simulink model "TP2_R3FOCPuente_ctrl_2016"  (R2016a)
settings: Solver=ode15s  StartTime=0.0  StopTime=.2  FixedStep=1e-6  RelTol=1e-5
values from neighbouring files (symbols this model uses):
  t1 = fase1+theta    (= 0.005)    [TP2_R3FMO_ctrl_2016.m]    (also in TP2_R3FMO_ctrl_2016_p_2.m; TP2_R3FMO_ctrl_2016_p_3.m)
  t2 = fase2+theta    (= 0.0116666666667)    [TP2_R3FMO_ctrl_2016.m]    (also in TP2_R3FMO_ctrl_2016_p_2.m; TP2_R3FMO_ctrl_2016_p_3.m)
  t3 = fase3+theta    (= 0.0183333333333)    [TP2_R3FMO_ctrl_2016.m]    (also in TP2_R3FMO_ctrl_2016_p_2.m; TP2_R3FMO_ctrl_2016_p_3.m)
undefined symbols (not defined in the file or in its folder): d
libraries: powerlib x21, powerlib_meascontrol x1
settings Model: Creator=Monina  LastModifiedBy=bress
settings DataIOCC: SaveFormat=Array  SignalLoggingSaveFormat=ModelDataLogs  TimeSaveName=t
settings OptimizationCC: ExpressionDepthLimit=2147483647
settings DebuggingCC: UnderspecifiedInitializationDetection=Classic  MergeDetectMultiDrivingBlocksExec=none  SolverPrmCheckMsg=warning  FcnCallInpInsideContextMsg=EnableAllAsWarning  StateNameClashWarn=warning
settings HardwareCC: ProdBitPerPointer=32  ProdLargestAtomicFloat=None  ProdIntDivRoundTo=Undefined  ProdEndianess=Unspecified  ProdWordSize=32  ProdHWDeviceType=32-bit Generic
settings ModelReferenceCC: PropagateSignalLabelsOutOfModel=off
settings GRTTargetCC: CombineOutputUpdateFcns=off  GRTInterface=on
settings ConfigComp: CovSFcnEnable=off
settings SimscapeCC: SimscapeNormalizeSystem=off

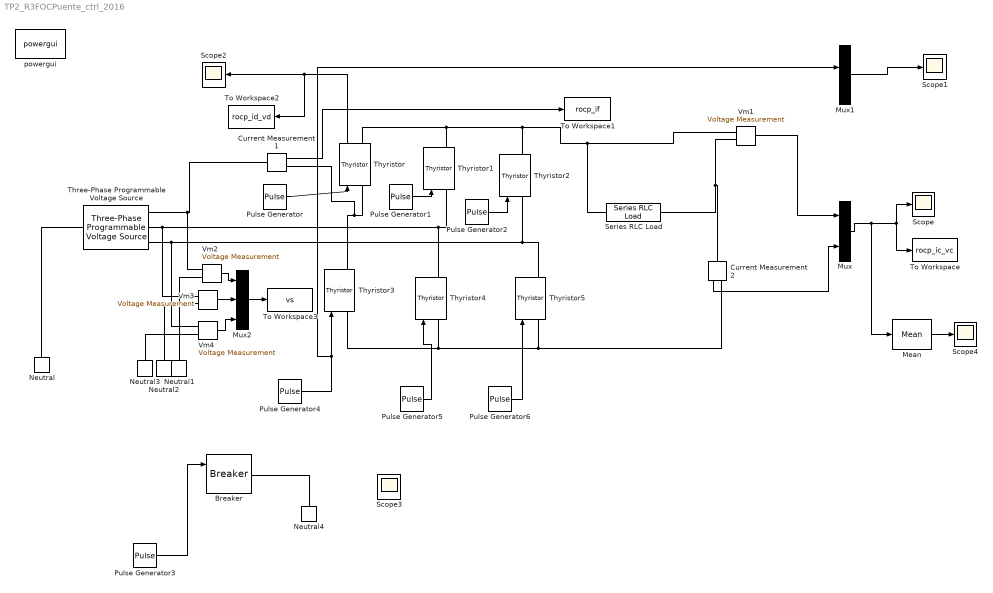
== system TP2_R3FOCPuente_ctrl_2016 ==
  Breaker : powerlib/Elements/Breaker  InitialState=0  SwitchingTimes="[1/60  5/60]"  External=on  BreakerResistance=0.01  SnubberResistance=1e6  SnubberCapacitance=inf  Measurements=None  MoreParameters=on  NoBreakLoop=off
  Current Measurement1 : powerlib/Measurements/Current Measurement  PhasorSimulation=off  OutputType=Complex  PSBequivalent=0
  Current Measurement2 : powerlib/Measurements/Current Measurement  PhasorSimulation=off  OutputType=Complex  PSBequivalent=0
  Mean : powerlib_meascontrol/Measurements/Mean  Freq=50  Vinit=0  Ts=0
  Mux : Mux  Inputs=2
  Mux1 : Mux
  Mux2 : Mux  Inputs=3
  Neutral{,1..4} (5 alike) : powerlib/Elements/Neutral  LConnTagsString=a  NodeNumber=10
  Pulse Generator : DiscretePulseGenerator  PulseType=Time based  Period=.02  PulseWidth=d  PhaseDelay=t1
  Pulse Generator1 : DiscretePulseGenerator  PulseType=Time based  Period=.02  PulseWidth=d  PhaseDelay=t2
  Pulse Generator2 : DiscretePulseGenerator  PulseType=Time based  Period=.02  PulseWidth=d  PhaseDelay=t3
  Pulse Generator3 : DiscretePulseGenerator  PulseType=Time based  Period=10  PulseWidth=50  PhaseDelay=.5
  Pulse Generator4 : DiscretePulseGenerator  PulseType=Time based  Period=.02  PulseWidth=d  PhaseDelay=t1+.01
  Pulse Generator5 : DiscretePulseGenerator  PulseType=Time based  Period=.02  PulseWidth=d  PhaseDelay=t2+.01
  Pulse Generator6 : DiscretePulseGenerator  PulseType=Time based  Period=.02  PulseWidth=d  PhaseDelay=t3+.01
  Scope{,1..4} (5 alike) : Scope
  Series RLC Load : powerlib/Elements/Series RLC Load  LConnTagsString=a  RConnTagsString=__new0  NominalVoltage=220  NominalFrequency=50  ActivePower=5000  InductivePower=500  CapacitivePower=0  Setx0=off  InitialVoltage=0  SetiL0=off  InitialCurrent=0  Measurements=None  LoadType=constant Z
  Three-Phase Programmable Voltage Source : powerlib/Electrical Sources/Three-Phase Programmable Voltage Source  PositiveSequence="[380  0 50]"  VariationEntity=None  VariationType=Table of time-amplitude pairs  VariationTypeAlt=Step  VariationStep=0.5  VariationRate=10  VariationMagnitude=0.3  VariationFrequency=2  VariationTiming=[1 2]  VariationPhaseA=off  Amplitudes=[1 0.8 1.2 1.0]  TimeValues=[0 0.1 0.15 0.2]  HarmonicGeneration=off  HarmonicA=[3 0.2 -25 0]  HarmonicB=[2 0.15 35 2]  Timing="[0.05  3]"  BusType=swing  Pref=0  Qref=0  Qmin=-inf  Qmax=inf
  Thyristor{,1..5} (6 alike) : powerlib/Power Electronics/Thyristor  Ron=0.001  Lon=0  Vf=0.8  IC=0  Rs=400  Cs=500e-10  Measurements=on
  To Workspace : ToWorkspace  VariableName=rocp_ic_vc  SampleTime=-1
  To Workspace1 : ToWorkspace  VariableName=rocp_if  SampleTime=-1
  To Workspace2 : ToWorkspace  VariableName=rocp_id_vd  SampleTime=-1
  To Workspace3 : ToWorkspace  VariableName=vs  SampleTime=-1
  Vm{1..4} (4 alike) : powerlib/Measurements/Voltage Measurement  PhasorSimulation=off  OutputType=Complex  PSBequivalent=0
  powergui : powerlib/powergui  Priority=1  SimulationMode=Continuous  SampleTime=50e-6  frequency=60  Iterations=50  frequencyindice=50  Pbase=100e6  ErrMax=1e-4  UnitsV=kV  UnitsW=MW  buscounter=0  FunctionMessages=off  echomessages=off  EnableUseOfTLC=off  CurrentSourceSwitches=on  DisableSnubberDevices=off  DisableRonSwitches=off  DisableVfSwitches=off  DisplayEquations=off  SolverType=Tustin  Interpol=off  ExternalGateDelay=off  methode=off  Ts=0  x0status=blocks  SPID=off  SwTol=0  HookPort=off  RestoreLinks=warning  ResistiveCurrentMeasurement=off  Frange=[0:2:500]  Ylog=off  Xlog=on  ShowGrid=off  save=off  variable=ZData  structure=0  ZoomFFT=off  StartTime=0.0  cycles=1  DisplayStyle=1  fundamental=60  FreqAxis=off  MaxFrequency=1000  frequencyindicesteady=1  RmsSteady=1  display=off
  wires:
  Mux/1 -> Mean/1, Scope/1, To Workspace/1
  Current Measurement1/1 -> To Workspace1/1
  Thyristor/1 -> To Workspace2/1, Scope2/1
  Mux1/1 -> Scope1/1
  Current Measurement2/1 -> Mux/2
  Pulse Generator/1 -> Thyristor/1
  Pulse Generator1/1 -> Thyristor1/1
  Pulse Generator2/1 -> Thyristor2/1
  Vm2/1 -> Mux2/1
  Vm3/1 -> Mux2/2
  Vm4/1 -> Mux2/3
  Mux2/1 -> To Workspace3/1
  Vm1/1 -> Mux/1
  Mean/1 -> Scope4/1
  Pulse Generator3/1 -> Breaker/1
  Pulse Generator4/1 -> Mux1/2, Thyristor3/1
  Pulse Generator5/1 -> Thyristor4/1
  Pulse Generator6/1 -> Thyristor5/1
  connections:
  Three-Phase Programmable Voltage Source/LConn1 -- Neutral/LConn1
  Series RLC Load/LConn1 -- Vm1/LConn1 -- Thyristor2/RConn1 -- Thyristor1/RConn1 -- Thyristor/RConn1
  Current Measurement2/RConn1 -- Thyristor3/LConn1 -- Thyristor4/LConn1 -- Thyristor5/LConn1
  Current Measurement1/RConn1 -- Thyristor3/RConn1 -- Thyristor/LConn1
  Current Measurement2/LConn1 -- Series RLC Load/RConn1 -- Vm1/LConn2
  Three-Phase Programmable Voltage Source/RConn2 -- Vm3/LConn1 -- Thyristor1/LConn1 -- Thyristor4/RConn1
  Three-Phase Programmable Voltage Source/RConn3 -- Vm4/LConn1 -- Thyristor2/LConn1 -- Thyristor5/RConn1
  Three-Phase Programmable Voltage Source/RConn1 -- Vm2/LConn1 -- Current Measurement1/LConn1
  Vm2/LConn2 -- Neutral1/LConn1
  Neutral2/LConn1 -- Vm3/LConn2
  Vm4/LConn2 -- Neutral3/LConn1
  Breaker/RConn1 -- Neutral4/LConn1
